simulink subsystem "IntersectionLogic"  (R2020a)
settings: Solver=VariableStepAuto  StartTime=0.0  StopTime=10.0  RelTol=1e-3
undefined symbols (not defined in the file or in its folder): num_signals
settings Model: Creator=frede  LastModifiedBy=zinoex

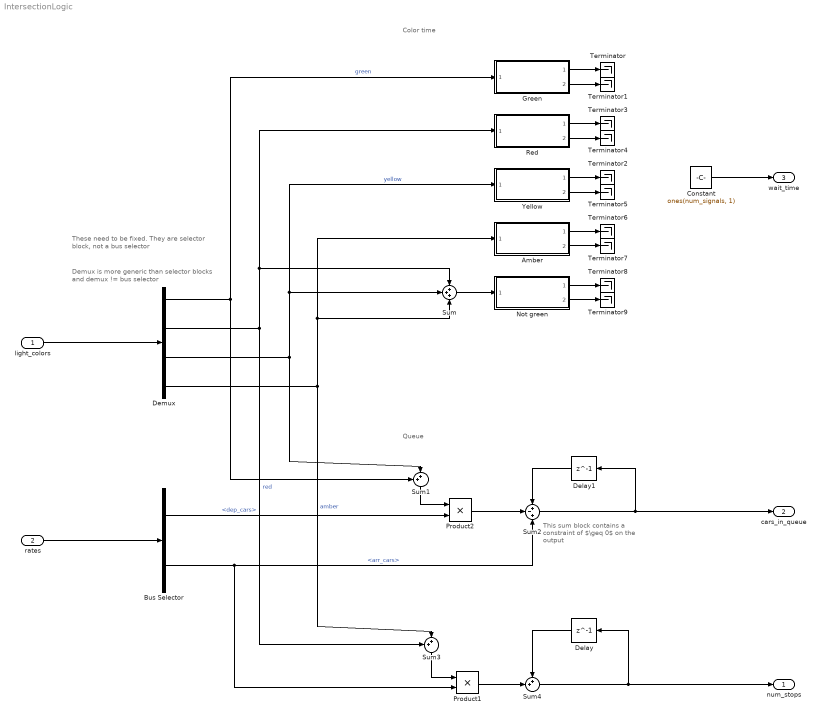
== system IntersectionLogic ==
  note: Demux is more generic than selector blocks
      | and demux != bus selector
  note: These need to be fixed.
      | They are selector block, not a bus selector
  note: This sum block contains a
      | constraint of $\geq 0$ on the output
  note: Queue
  note: Color time
  light_colors : Inport
  rates : Inport  Port=2
  Amber : Subsystem  ReferencedSubsystem=Timer
  Bus Selector : BusSelector  OutputSignals=dep_cars,arr_cars
  Constant : Constant  Value=ones(num_signals, 1)
  Delay : Delay  DelayLength=1
  Delay1 : Delay  DelayLength=1
  Demux : Demux
  Green : Subsystem  ReferencedSubsystem=Timer
  Not green : Subsystem  ReferencedSubsystem=Timer
  Product1 : Product
  Product2 : Product
  Red : Subsystem  ReferencedSubsystem=Timer
  Sum : Sum  Inputs=+++
  Sum1 : Sum  Inputs=++|
  Sum2 : Sum  Inputs=+-+  OutMin=0
  Sum3 : Sum  Inputs=++|
  Sum4 : Sum  Inputs=++|
  Terminator{,1..9} (10 alike) : Terminator
  Yellow : Subsystem  ReferencedSubsystem=Timer
  num_stops : Outport
  cars_in_queue : Outport  Port=2
  wait_time : Outport  Port=3
  wires:
  rates/1 -> Bus Selector/1
  Demux/2 -> Sum3/1, Red/1, Sum/1  "red"
  Demux/4 -> Sum3/2, Amber/1, Sum/3  "amber"
  Demux/3 -> Sum/2, Yellow/1, Sum1/2  "yellow"
  Demux/1 -> Green/1, Sum1/1  "green"
  Sum/1 -> Not green/1
  Bus Selector/2 -> Product1/2, Sum2/3  "<arr_cars>"
  Sum3/1 -> Product1/1
  Product1/1 -> Sum4/2
  Delay/1 -> Sum4/1
  Sum4/1 -> num_stops/1, Delay/1
  Sum2/1 -> cars_in_queue/1, Delay1/1
  Constant/1 -> wait_time/1
  light_colors/1 -> Demux/1
  Not green/1 -> Terminator8/1
  Not green/2 -> Terminator9/1
  Amber/1 -> Terminator6/1
  Amber/2 -> Terminator7/1
  Yellow/2 -> Terminator5/1
  Yellow/1 -> Terminator2/1
  Red/2 -> Terminator4/1
  Red/1 -> Terminator3/1
  Green/2 -> Terminator1/1
  Green/1 -> Terminator/1
  Delay1/1 -> Sum2/1
  Bus Selector/1 -> Product2/2  "<dep_cars>"
  Sum1/1 -> Product2/1
  Product2/1 -> Sum2/2
